simulink model "Simulink_DiscoRotante"  (R2025b)
settings: Solver=ode45  StartTime=0.0  StopTime=10.0  MaxStep=0.001  RelTol=1e-3
values from neighbouring files (symbols this model uses):
  k = 100    [DiscoRodante.m]
  m = 10    [DiscoRodante.m]
settings Model: Creator=Valeria Mar  LastModifiedBy=Valeria Mar

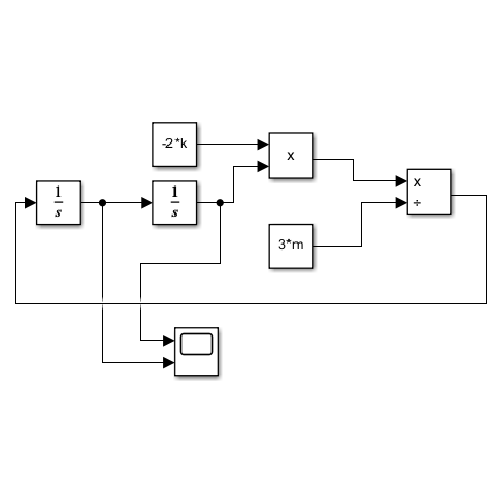
[thumbnail: Simulink's stored preview of the top-level diagram]
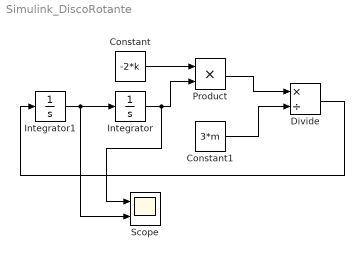
== system Simulink_DiscoRotante ==
  Constant : Constant  Value=-2*k
  Constant1 : Constant  Value=3*m
  Divide : Product  Inputs=*/
  Integrator : Integrator
  Integrator1 : Integrator  InitialCondition=2
  Product : Product
  Scope : Scope  NumInputPorts=2
      settings: ActiveDisplayYMinimum=-2.499549387411887  ActiveDisplayYMaximum=2.4999499319346539
  wires:
  Constant/1 -> Product/1
  Integrator/1 -> Scope/1, Product/2
  Product/1 -> Divide/1
  Constant1/1 -> Divide/2
  Integrator1/1 -> Scope/2, Integrator/1
  Divide/1 -> Integrator1/1
